simulink model "FIR_Filter"  (R2023b)
settings: Solver=FixedStepDiscrete  StartTime=0.0  StopTime=0.01  RelTol=1e-3
PreLoadFcn:
  | addpath('D:\Digital IC\FPGA\fir_filter\verif\hdlimport\FIR_Filter');
libraries: hdlmdlgenlib x60, dspsrcs4 x2
CloseFcn:
  | addpath('D:\Digital IC\FPGA\fir_filter\verif\hdlimport\FIR_Filter');
  | rmpath('D:\Digital IC\FPGA\fir_filter\verif\hdlimport\FIR_Filter');
settings Model: DataTypeOverride=Off  Creator=Abanoub Hanna  LastModifiedBy=Abanoub Hanna
settings OptimizationCC: BlockReduction=off  ConditionallyExecuteInputs=off  DefaultParameterBehavior=Inlined  InheritOutputTypeSmallerThanSingle=on
settings DebuggingCC: AlgebraicLoopMsg=error  InheritedTsInSrcMsg=none  SingleTaskRateTransMsg=error  ParameterPrecisionLossMsg=none
settings HardwareCC: ProdBitPerPointer=32  ProdBitPerSizeT=32  ProdBitPerPtrDiffT=32  ProdLargestAtomicFloat=None  ProdIntDivRoundTo=Undefined  ProdEndianess=Unspecified  ProdWordSize=32  ProdHWDeviceType=ASIC/FPGA->ASIC/FPGA  TargetBitPerPointer=64  TargetBitPerSizeT=64  TargetBitPerPtrDiffT=64  TargetLongLongMode=on  TargetIntDivRoundTo=Zero  TargetEndianess=LittleEndian  TargetWordSize=64  TargetHWDeviceType=Custom Processor->MATLAB Host Computer  ProdEqTarget=off

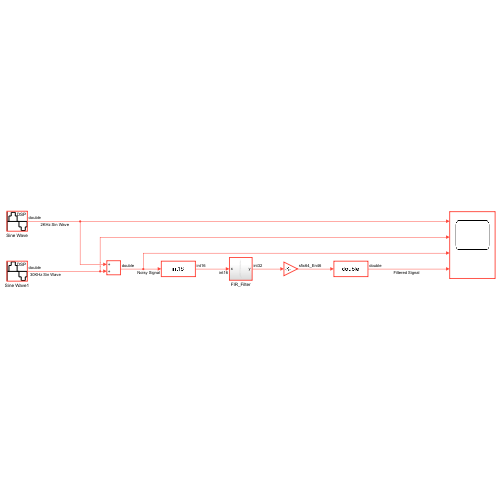
[thumbnail: Simulink's stored preview of the top-level diagram]
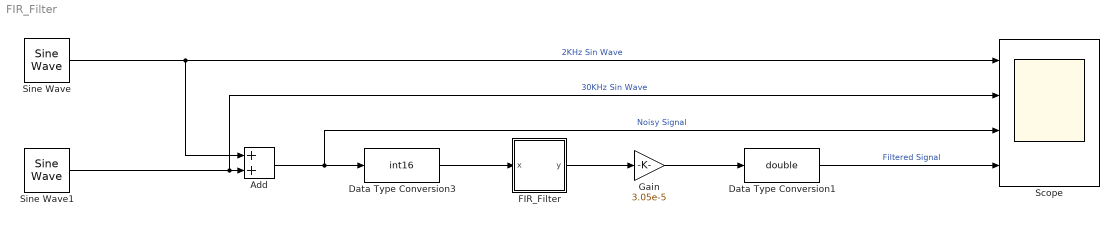
== system FIR_Filter ==
  Add : Sum  OutDataTypeStr=double
  Data Type Conversion1 : DataTypeConversion  OutDataTypeStr=double  RndMeth=Round  SaturateOnIntegerOverflow=off
  Data Type Conversion3 : DataTypeConversion  OutDataTypeStr=int16  RndMeth=Round  SaturateOnIntegerOverflow=off
  FIR_Filter : Subsystem
  Gain : Gain  Gain=3.05e-5
  Scope : Scope  NumInputPorts=4
  Sine Wave : dspsrcs4/Sine Wave  Amplitude=1  Frequency=2000  Phase=0  SampleMode=Discrete  OutComplex=Real  CompMethod=Trigonometric fcn  TableSize=Speed  SampleTime=1/100000  SamplesPerFrame=1  ResetState=Restart at time zero  OutputFrames=off  dataType=double  wordLen=16  udDataType=sfix(16)  fracBitsMode=Best precision  numFracBits=15  OutDataTypeStr=double  LastOutDataTypeStr=double
  Sine Wave1 : dspsrcs4/Sine Wave  Amplitude=1  Frequency=30000  Phase=0  SampleMode=Discrete  OutComplex=Real  CompMethod=Trigonometric fcn  TableSize=Speed  SampleTime=1/100000  SamplesPerFrame=1  ResetState=Restart at time zero  OutputFrames=off  dataType=double  wordLen=16  udDataType=sfix(16)  fracBitsMode=Best precision  numFracBits=15  OutDataTypeStr=double  LastOutDataTypeStr=double
  wires:
  Sine Wave/1 -> Add/1, Scope/1  "2KHz Sin Wave"
  Add/1 -> Scope/3, Data Type Conversion3/1  "Noisy Signal"
  FIR_Filter/1(y) -> Gain/1
  Gain/1 -> Data Type Conversion1/1
  Data Type Conversion3/1 -> FIR_Filter/1(x)
  Data Type Conversion1/1 -> Scope/4  "Filtered Signal"
  Sine Wave1/1 -> Scope/2, Add/2  "30KHz Sin Wave"

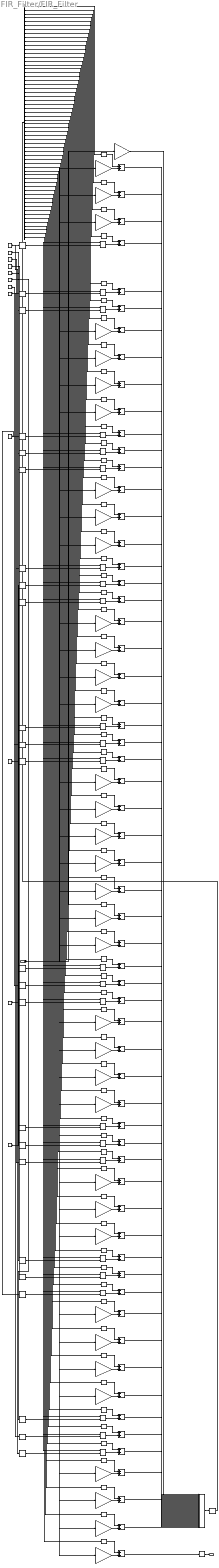
== system FIR_Filter/FIR_Filter ==
  x : Inport  OutDataTypeStr=int16  SampleTime=-1
  Add : Sum  OutDataTypeStr=int32  AccumDataTypeStr=int32  SampleTime=-1
  Add_{1..59} (59 alike) : Sum  OutDataTypeStr=int32  AccumDataTypeStr=int32  SampleTime=-1
  CONST_s32b_1479 : Constant  Value=1479  OutDataTypeStr=int32  SampleTime=-1
  CONST_s32b_168 : Constant  Value=168  OutDataTypeStr=int32  SampleTime=-1
  CONST_s32b_184 : Constant  Value=184  OutDataTypeStr=int32  SampleTime=-1
  CONST_s32b_1973 : Constant  Value=1973  OutDataTypeStr=int32  SampleTime=-1
  CONST_s32b_252 : Constant  Value=252  OutDataTypeStr=int32  SampleTime=-1
  CONST_s32b_36 : Constant  Value=36  OutDataTypeStr=int32  SampleTime=-1
  CONST_s32b_55 : Constant  Value=55  OutDataTypeStr=int32  SampleTime=-1
  CONST_s32b_582 : Constant  Value=582  OutDataTypeStr=int32  SampleTime=-1
  CONST_s32b_594 : Constant  Value=594  OutDataTypeStr=int32  SampleTime=-1
  CONST_s32b_77 : Constant  Value=77  OutDataTypeStr=int32  SampleTime=-1
  CONST_s32b_943 : Constant  Value=943  OutDataTypeStr=int32  SampleTime=-1
  CONST_s32b_95 : Constant  Value=95  OutDataTypeStr=int32  SampleTime=-1
  Mul{79,127,559,607} (4 alike) : Gain  Gain="fi(0,1,32,0,\"hex\",\"00000023\")"  ParamDataTypeStr=fixdt(1, 32, 0)  OutDataTypeStr=int32  SampleTime=-1
  Mul136 : Gain  Gain="fi(0,1,32,0,\"hex\",\"00000083\")"  ParamDataTypeStr=fixdt(1, 32, 0)  OutDataTypeStr=int32  SampleTime=-1
  Mul145 : Gain  Gain="fi(0,1,32,0,\"hex\",\"00000085\")"  ParamDataTypeStr=fixdt(1, 32, 0)  OutDataTypeStr=int32  SampleTime=-1
  Mul{62,154,250,436,532,624} (6 alike) : Gain  Gain="fi(0,1,32,0,\"hex\",\"00000000\")"  ParamDataTypeStr=fixdt(1, 32, 0)  OutDataTypeStr=int32  SampleTime=-1
  Mul193 : Gain  Gain="fi(0,1,32,0,\"hex\",\"000000d1\")"  ParamDataTypeStr=fixdt(1, 32, 0)  OutDataTypeStr=int32  SampleTime=-1
  Mul202 : Gain  Gain="fi(0,1,32,0,\"hex\",\"0000019a\")"  ParamDataTypeStr=fixdt(1, 32, 0)  OutDataTypeStr=int32  SampleTime=-1
  Mul211 : Gain  Gain="fi(0,1,32,0,\"hex\",\"00000115\")"  ParamDataTypeStr=fixdt(1, 32, 0)  OutDataTypeStr=int32  SampleTime=-1
  Mul259 : Gain  Gain="fi(0,1,32,0,\"hex\",\"0000030d\")"  ParamDataTypeStr=fixdt(1, 32, 0)  OutDataTypeStr=int32  SampleTime=-1
  Mul268 : Gain  Gain="fi(0,1,32,0,\"hex\",\"00000432\")"  ParamDataTypeStr=fixdt(1, 32, 0)  OutDataTypeStr=int32  SampleTime=-1
  Mul277 : Gain  Gain="fi(0,1,32,0,\"hex\",\"0000019d\")"  ParamDataTypeStr=fixdt(1, 32, 0)  OutDataTypeStr=int32  SampleTime=-1
  Mul316 : Gain  Gain="fi(0,1,32,0,\"hex\",\"0000041d\")"  ParamDataTypeStr=fixdt(1, 32, 0)  OutDataTypeStr=int32  SampleTime=-1
  Mul325 : Gain  Gain="fi(0,1,32,0,\"hex\",\"00001334\")"  ParamDataTypeStr=fixdt(1, 32, 0)  OutDataTypeStr=int32  SampleTime=-1
  Mul334 : Gain  Gain="fi(0,1,32,0,\"hex\",\"000020e4\")"  ParamDataTypeStr=fixdt(1, 32, 0)  OutDataTypeStr=int32  SampleTime=-1
  Mul343 : Gain  Gain="fi(0,1,32,0,\"hex\",\"00002666\")"  ParamDataTypeStr=fixdt(1, 32, 0)  OutDataTypeStr=int32  SampleTime=-1
  Mul352 : Gain  Gain="fi(0,1,32,0,\"hex\",\"000020e4\")"  ParamDataTypeStr=fixdt(1, 32, 0)  OutDataTypeStr=int32  SampleTime=-1
  Mul361 : Gain  Gain="fi(0,1,32,0,\"hex\",\"00001334\")"  ParamDataTypeStr=fixdt(1, 32, 0)  OutDataTypeStr=int32  SampleTime=-1
  Mul370 : Gain  Gain="fi(0,1,32,0,\"hex\",\"0000041d\")"  ParamDataTypeStr=fixdt(1, 32, 0)  OutDataTypeStr=int32  SampleTime=-1
  Mul409 : Gain  Gain="fi(0,1,32,0,\"hex\",\"0000019d\")"  ParamDataTypeStr=fixdt(1, 32, 0)  OutDataTypeStr=int32  SampleTime=-1
  Mul418 : Gain  Gain="fi(0,1,32,0,\"hex\",\"00000432\")"  ParamDataTypeStr=fixdt(1, 32, 0)  OutDataTypeStr=int32  SampleTime=-1
  Mul427 : Gain  Gain="fi(0,1,32,0,\"hex\",\"0000030d\")"  ParamDataTypeStr=fixdt(1, 32, 0)  OutDataTypeStr=int32  SampleTime=-1
  Mul475 : Gain  Gain="fi(0,1,32,0,\"hex\",\"00000115\")"  ParamDataTypeStr=fixdt(1, 32, 0)  OutDataTypeStr=int32  SampleTime=-1
  Mul484 : Gain  Gain="fi(0,1,32,0,\"hex\",\"0000019a\")"  ParamDataTypeStr=fixdt(1, 32, 0)  OutDataTypeStr=int32  SampleTime=-1
  Mul493 : Gain  Gain="fi(0,1,32,0,\"hex\",\"000000d1\")"  ParamDataTypeStr=fixdt(1, 32, 0)  OutDataTypeStr=int32  SampleTime=-1
  Mul541 : Gain  Gain="fi(0,1,32,0,\"hex\",\"00000085\")"  ParamDataTypeStr=fixdt(1, 32, 0)  OutDataTypeStr=int32  SampleTime=-1
  Mul550 : Gain  Gain="fi(0,1,32,0,\"hex\",\"00000083\")"  ParamDataTypeStr=fixdt(1, 32, 0)  OutDataTypeStr=int32  SampleTime=-1
  Mul598 : Gain  Gain="fi(0,1,32,0,\"hex\",\"0000000f\")"  ParamDataTypeStr=fixdt(1, 32, 0)  OutDataTypeStr=int32  SampleTime=-1
  Mul616 : Gain  Gain="fi(0,1,32,0,\"hex\",\"00000016\")"  ParamDataTypeStr=fixdt(1, 32, 0)  OutDataTypeStr=int32  SampleTime=-1
  Mul70 : Gain  Gain="fi(0,1,32,0,\"hex\",\"00000016\")"  ParamDataTypeStr=fixdt(1, 32, 0)  OutDataTypeStr=int32  SampleTime=-1
  Mul88 : Gain  Gain="fi(0,1,32,0,\"hex\",\"0000000f\")"  ParamDataTypeStr=fixdt(1, 32, 0)  OutDataTypeStr=int32  SampleTime=-1
  Mul_{4..6,11..13,17..19,24..26,34..36,41..43,47..49,54..56} (24 alike) : Product  Inputs=**  OutDataTypeStr=int32  SampleTime=-1
  Uminus : UnaryMinus  SampleTime=-1
  Uminus_{1..23} (23 alike) : UnaryMinus  SampleTime=-1
  VectorConcat : Concatenate  NumInputs=60
  acc_FF_0_wire : hdlmdlgenlib/Buffer
  acc_FF_10_wire : hdlmdlgenlib/Buffer
  acc_FF_11_wire : hdlmdlgenlib/Buffer
  acc_FF_12_wire : hdlmdlgenlib/Buffer
  acc_FF_13_wire : hdlmdlgenlib/Buffer
  acc_FF_14_wire : hdlmdlgenlib/Buffer
  acc_FF_15_wire : hdlmdlgenlib/Buffer
  acc_FF_16_wire : hdlmdlgenlib/Buffer
  acc_FF_17_wire : hdlmdlgenlib/Buffer
  acc_FF_18_wire : hdlmdlgenlib/Buffer
  acc_FF_19_wire : hdlmdlgenlib/Buffer
  acc_FF_1_wire : hdlmdlgenlib/Buffer
  acc_FF_20_wire : hdlmdlgenlib/Buffer
  acc_FF_21_wire : hdlmdlgenlib/Buffer
  acc_FF_22_wire : hdlmdlgenlib/Buffer
  acc_FF_23_wire : hdlmdlgenlib/Buffer
  acc_FF_24_wire : hdlmdlgenlib/Buffer
  acc_FF_25_wire : hdlmdlgenlib/Buffer
  acc_FF_26_wire : hdlmdlgenlib/Buffer
  acc_FF_27_wire : hdlmdlgenlib/Buffer
  acc_FF_28_wire : hdlmdlgenlib/Buffer
  acc_FF_29_wire : hdlmdlgenlib/Buffer
  acc_FF_2_wire : hdlmdlgenlib/Buffer
  acc_FF_30_wire : hdlmdlgenlib/Buffer
  acc_FF_31_wire : hdlmdlgenlib/Buffer
  acc_FF_32_wire : hdlmdlgenlib/Buffer
  acc_FF_33_wire : hdlmdlgenlib/Buffer
  acc_FF_34_wire : hdlmdlgenlib/Buffer
  acc_FF_35_wire : hdlmdlgenlib/Buffer
  acc_FF_36_wire : hdlmdlgenlib/Buffer
  acc_FF_37_wire : hdlmdlgenlib/Buffer
  acc_FF_38_wire : hdlmdlgenlib/Buffer
  acc_FF_39_wire : hdlmdlgenlib/Buffer
  acc_FF_3_wire : hdlmdlgenlib/Buffer
  acc_FF_40_wire : hdlmdlgenlib/Buffer
  acc_FF_41_wire : hdlmdlgenlib/Buffer
  acc_FF_42_wire : hdlmdlgenlib/Buffer
  acc_FF_43_wire : hdlmdlgenlib/Buffer
  acc_FF_44_wire : hdlmdlgenlib/Buffer
  acc_FF_45_wire : hdlmdlgenlib/Buffer
  acc_FF_46_wire : hdlmdlgenlib/Buffer
  acc_FF_47_wire : hdlmdlgenlib/Buffer
  acc_FF_48_wire : hdlmdlgenlib/Buffer
  acc_FF_49_wire : hdlmdlgenlib/Buffer
  acc_FF_4_wire : hdlmdlgenlib/Buffer
  acc_FF_50_wire : hdlmdlgenlib/Buffer
  acc_FF_51_wire : hdlmdlgenlib/Buffer
  acc_FF_52_wire : hdlmdlgenlib/Buffer
  acc_FF_53_wire : hdlmdlgenlib/Buffer
  acc_FF_54_wire : hdlmdlgenlib/Buffer
  acc_FF_55_wire : hdlmdlgenlib/Buffer
  acc_FF_56_wire : hdlmdlgenlib/Buffer
  acc_FF_57_wire : hdlmdlgenlib/Buffer
  acc_FF_58_wire : hdlmdlgenlib/Buffer
  acc_FF_59_wire : hdlmdlgenlib/Buffer
  acc_FF_5_wire : hdlmdlgenlib/Buffer
  acc_FF_6_wire : hdlmdlgenlib/Buffer
  acc_FF_7_wire : hdlmdlgenlib/Buffer
  acc_FF_8_wire : hdlmdlgenlib/Buffer
  acc_FF_9_wire : hdlmdlgenlib/Buffer
  acc_reg : Delay  DelayLength=double(1)  InitialCondition=0  SampleTime=-1
  t : Demux  Outputs=60
  y_1_reg : Delay  DelayLength=double(1)  InitialCondition=0  SampleTime=-1
  y : Outport  OutDataTypeStr=int32  SampleTime=-1
  wires:
  t/2 -> acc_FF_1_wire/1
  Mul_41/1 -> Add_40/2
  t/56 -> acc_FF_55_wire/1
  Add_25/1 -> VectorConcat/27
  acc_FF_32_wire/1 -> Add_32/1
  t/57 -> acc_FF_56_wire/1
  Uminus_18/1 -> Mul_47/2
  Mul418/1 -> Add_37/2
  Add_54/1 -> VectorConcat/56
  Mul_25/1 -> Add_24/2
  t/10 -> acc_FF_9_wire/1
  acc_FF_47_wire/1 -> Add_47/1
  Add_10/1 -> VectorConcat/12
  Mul277/1 -> Add_22/2
  t/59 -> acc_FF_58_wire/1
  t/4 -> acc_FF_3_wire/1
  Mul624/1 -> Add_59/2
  t/52 -> acc_FF_51_wire/1
  t/3 -> acc_FF_2_wire/1
  t/58 -> acc_FF_57_wire/1
  t/60 -> acc_FF_59_wire/1
  Mul_49/1 -> Add_48/2
  t/5 -> acc_FF_4_wire/1
  acc_FF_59_wire/1 -> Add_59/1
  CONST_s32b_36/1 -> Uminus/1, Uminus_23/1
  Add_13/1 -> VectorConcat/15
  t/18 -> acc_FF_17_wire/1
  Add_58/1 -> VectorConcat/60
  t/54 -> acc_FF_53_wire/1
  t/1 -> acc_FF_0_wire/1
  CONST_s32b_55/1 -> Uminus_21/1, Uminus_2/1
  t/55 -> acc_FF_54_wire/1
  Mul343/1 -> Add_29/2
  t/53 -> acc_FF_52_wire/1
  acc_FF_9_wire/1 -> Add_9/1
  Mul370/1 -> Add_32/2
  acc_FF_39_wire/1 -> Add_39/1
  Mul_18/1 -> Add_17/2
  t/35 -> acc_FF_34_wire/1
  Mul334/1 -> Add_28/2
  acc_FF_41_wire/1 -> Add_41/1
  t/51 -> acc_FF_50_wire/1
  Add_26/1 -> VectorConcat/28
  acc_reg/1 -> t/1
  Mul_56/1 -> Add_55/2
  x/1 -> Mul62/1, Mul624/1, Mul616/1, Mul_55/1, Mul_54/1, Mul541/1, Mul532/1, Mul475/1, Mul_43/1, Mul559/1, Mul436/1, Mul427/1, Mul409/1, Mul_36/1, Mul_34/1, Mul370/1, Mul_48/1, Mul361/1, Mul352/1, Mul343/1, Mul325/1, Mul316/1, Mul_26/1, Mul_25/1, Mul_24/1, Mul268/1, Mul259/1, Mul250/1, Mul_19/1, Mul_18/1, Mul_17/1, Mul211/1, Mul202/1, Mul193/1, Mul_12/1, Mul_11/1, Mul145/1, Mul127/1, Mul_6/1, Mul_5/1, Mul_4/1, Mul88/1, Mul79/1, Mul70/1, Mul607/1, Mul550/1, Mul_56/1, Mul_41/1, Mul154/1, Mul484/1, Mul_47/1, Mul277/1, Mul598/1, Mul_42/1, Mul334/1, Mul136/1, Mul493/1, Mul_49/1, Mul_13/1, Mul_35/1, Mul418/1
  Add_44/1 -> VectorConcat/46
  acc_FF_24_wire/1 -> Add_24/1
  Uminus_4/1 -> Mul_12/2
  Uminus_11/1 -> Mul_26/2
  t/50 -> acc_FF_49_wire/1
  t/48 -> acc_FF_47_wire/1
  t/49 -> acc_FF_48_wire/1
  t/47 -> acc_FF_46_wire/1
  Add_57/1 -> VectorConcat/59
  Add_16/1 -> VectorConcat/18
  CONST_s32b_943/1 -> Uminus_9/1, Uminus_14/1
  t/7 -> acc_FF_6_wire/1
  Uminus_6/1 -> Mul_17/2
  t/46 -> acc_FF_45_wire/1
  acc_FF_43_wire/1 -> Add_43/1
  t/19 -> acc_FF_18_wire/1
  Mul_42/1 -> Add_41/2
  t/34 -> acc_FF_33_wire/1
  acc_FF_30_wire/1 -> Add_30/1
  t/45 -> acc_FF_44_wire/1
  Add_8/1 -> VectorConcat/10
  t/44 -> acc_FF_43_wire/1
  t/42 -> acc_FF_41_wire/1
  acc_FF_46_wire/1 -> Add_46/1
  Uminus_13/1 -> Mul_35/2
  Mul475/1 -> Add_43/2
  t/43 -> acc_FF_42_wire/1
  Mul_4/1 -> Add_3/2
  t/41 -> acc_FF_40_wire/1
  CONST_s32b_1479/1 -> Uminus_12/1, Uminus_11/1
  Mul70/1 -> Add/2
  t/40 -> acc_FF_39_wire/1
  Mul259/1 -> Add_20/2
  t/39 -> acc_FF_38_wire/1
  t/38 -> acc_FF_37_wire/1
  t/37 -> acc_FF_36_wire/1
  Uminus/1 -> Mul_4/2
  t/36 -> acc_FF_35_wire/1
  acc_FF_35_wire/1 -> Add_35/1
  Uminus_15/1 -> Mul_41/2
  t/9 -> acc_FF_8_wire/1
  CONST_s32b_594/1 -> Uminus_16/1, Uminus_7/1
  t/25 -> acc_FF_24_wire/1
  y_1_reg/1 -> y/1
  Add_43/1 -> VectorConcat/45
  t/33 -> acc_FF_32_wire/1
  t/20 -> acc_FF_19_wire/1
  t/32 -> acc_FF_31_wire/1
  t/31 -> acc_FF_30_wire/1
  t/27 -> acc_FF_26_wire/1
  Add_12/1 -> VectorConcat/14
  t/30 -> acc_FF_29_wire/1
  t/29 -> acc_FF_28_wire/1
  t/28 -> acc_FF_27_wire/1
  t/21 -> acc_FF_20_wire/1
  t/24 -> acc_FF_23_wire/1
  Add_2/1 -> VectorConcat/4
  t/26 -> acc_FF_25_wire/1
  t/23 -> acc_FF_22_wire/1
  acc_FF_49_wire/1 -> Add_49/1
  Add/1 -> VectorConcat/2
  CONST_s32b_184/1 -> Uminus_20/1, Uminus_3/1
  acc_FF_13_wire/1 -> Add_13/1
  t/22 -> acc_FF_21_wire/1
  t/6 -> acc_FF_5_wire/1
  Add_37/1 -> VectorConcat/39
  t/15 -> acc_FF_14_wire/1
  t/17 -> acc_FF_16_wire/1
  t/16 -> acc_FF_15_wire/1
  acc_FF_55_wire/1 -> Add_55/1
  t/14 -> acc_FF_13_wire/1
  Add_22/1 -> VectorConcat/24
  t/13 -> acc_FF_12_wire/1
  t/12 -> acc_FF_11_wire/1
  t/11 -> acc_FF_10_wire/1
  Mul202/1 -> Add_14/2
  t/8 -> acc_FF_7_wire/1
  Add_59/1 -> y_1_reg/1
  Mul616/1 -> Add_58/2
  acc_FF_22_wire/1 -> Add_22/1
  Mul_34/1 -> Add_33/2
  Mul_26/1 -> Add_25/2
  Mul_12/1 -> Add_11/2
  Mul607/1 -> Add_57/2
  Add_56/1 -> VectorConcat/58
  Mul_55/1 -> Add_54/2
  Add_35/1 -> VectorConcat/37
  Mul598/1 -> Add_56/2
  Add_55/1 -> VectorConcat/57
  Mul532/1 -> Add_49/2
  Uminus_23/1 -> Mul_56/2
  Uminus_22/1 -> Mul_55/2
  Add_53/1 -> VectorConcat/55
  Mul_54/1 -> Add_53/2
  Uminus_21/1 -> Mul_54/2
  Uminus_14/1 -> Mul_36/2
  Add_52/1 -> VectorConcat/54
  acc_FF_31_wire/1 -> Add_31/1
  Mul559/1 -> Add_52/2
  Add_51/1 -> VectorConcat/53
  Mul_43/1 -> Add_42/2
  Mul550/1 -> Add_51/2
  Add_50/1 -> VectorConcat/52
  acc_FF_29_wire/1 -> Add_29/1
  Mul541/1 -> Add_50/2
  Add_49/1 -> VectorConcat/51
  Add_48/1 -> VectorConcat/50
  CONST_s32b_252/1 -> Uminus_4/1, Uminus_19/1
  Uminus_20/1 -> Mul_49/2
  Add_47/1 -> VectorConcat/49
  Mul_48/1 -> Add_47/2
  acc_FF_52_wire/1 -> Add_52/1
  Uminus_19/1 -> Mul_48/2
  Add_46/1 -> VectorConcat/48
  Mul_47/1 -> Add_46/2
  Add_45/1 -> VectorConcat/47
  Mul493/1 -> Add_45/2
  acc_FF_28_wire/1 -> Add_28/1
  Mul484/1 -> Add_44/2
  Uminus_3/1 -> Mul_11/2
  Add_42/1 -> VectorConcat/44
  Uminus_17/1 -> Mul_43/2
  Add_41/1 -> VectorConcat/43
  Uminus_16/1 -> Mul_42/2
  acc_FF_51_wire/1 -> Add_51/1
  Add_40/1 -> VectorConcat/42
  Add_39/1 -> VectorConcat/41
  acc_FF_21_wire/1 -> Add_21/1
  Mul436/1 -> Add_39/2
  Mul_17/1 -> Add_16/2
  Add_38/1 -> VectorConcat/40
  acc_FF_33_wire/1 -> Add_33/1
  Mul427/1 -> Add_38/2
  Add_36/1 -> VectorConcat/38
  Mul409/1 -> Add_36/2
  Mul_36/1 -> Add_35/2
  acc_FF_8_wire/1 -> Add_8/1
  Add_34/1 -> VectorConcat/36
  Mul_35/1 -> Add_34/2
  Add_33/1 -> VectorConcat/35
  Uminus_12/1 -> Mul_34/2
  Add_32/1 -> VectorConcat/34
  Add_31/1 -> VectorConcat/33
  Mul361/1 -> Add_31/2
  Add_30/1 -> VectorConcat/32
  acc_FF_2_wire/1 -> Add_2/1
  Mul352/1 -> Add_30/2
  Add_29/1 -> VectorConcat/31
  Add_28/1 -> VectorConcat/30
  Add_27/1 -> VectorConcat/29
  Mul325/1 -> Add_27/2
  Mul316/1 -> Add_26/2
  Mul88/1 -> Add_2/2
  Add_14/1 -> VectorConcat/16
  Add_24/1 -> VectorConcat/26
  Uminus_10/1 -> Mul_25/2
  Mul127/1 -> Add_6/2
  Mul145/1 -> Add_8/2
  Add_23/1 -> VectorConcat/25
  Mul_24/1 -> Add_23/2
  Uminus_9/1 -> Mul_24/2
  acc_FF_54_wire/1 -> Add_54/1
  Add_21/1 -> VectorConcat/23
  Mul268/1 -> Add_21/2
  Add_20/1 -> VectorConcat/22
  Add_19/1 -> VectorConcat/21
  Mul250/1 -> Add_19/2
  Add_18/1 -> VectorConcat/20
  Mul211/1 -> Add_15/2
  Mul_19/1 -> Add_18/2
  Uminus_8/1 -> Mul_19/2
  Add_17/1 -> VectorConcat/19
  Uminus_7/1 -> Mul_18/2
  acc_FF_36_wire/1 -> Add_36/1
  Add_15/1 -> VectorConcat/17
  CONST_s32b_582/1 -> Uminus_8/1, Uminus_15/1
  Mul193/1 -> Add_13/2
  Mul_13/1 -> Add_12/2
  VectorConcat/1 -> acc_reg/1
  Uminus_5/1 -> Mul_13/2
  CONST_s32b_95/1 -> Uminus_5/1, Uminus_18/1
  Add_11/1 -> VectorConcat/13
  Add_3/1 -> VectorConcat/5
  Mul_11/1 -> Add_10/2
  Add_9/1 -> VectorConcat/11
  Mul62/1 -> VectorConcat/1
  Mul154/1 -> Add_9/2
  CONST_s32b_1973/1 -> Uminus_10/1, Uminus_13/1
  Add_7/1 -> VectorConcat/9
  Mul136/1 -> Add_7/2
  Add_6/1 -> VectorConcat/8
  Add_5/1 -> VectorConcat/7
  Mul_6/1 -> Add_5/2
  Uminus_2/1 -> Mul_6/2
  Add_4/1 -> VectorConcat/6
  Mul_5/1 -> Add_4/2
  Uminus_1/1 -> Mul_5/2
  Add_1/1 -> VectorConcat/3
  Mul79/1 -> Add_1/2
  acc_FF_58_wire/1 -> Add_58/1
  acc_FF_57_wire/1 -> Add_57/1
  acc_FF_56_wire/1 -> Add_56/1
  acc_FF_53_wire/1 -> Add_53/1
  acc_FF_50_wire/1 -> Add_50/1
  acc_FF_48_wire/1 -> Add_48/1
  acc_FF_45_wire/1 -> Add_45/1
  acc_FF_44_wire/1 -> Add_44/1
  acc_FF_42_wire/1 -> Add_42/1
  acc_FF_40_wire/1 -> Add_40/1
  acc_FF_38_wire/1 -> Add_38/1
  acc_FF_18_wire/1 -> Add_18/1
  acc_FF_37_wire/1 -> Add_37/1
  acc_FF_34_wire/1 -> Add_34/1
  acc_FF_7_wire/1 -> Add_7/1
  acc_FF_27_wire/1 -> Add_27/1
  acc_FF_26_wire/1 -> Add_26/1
  acc_FF_25_wire/1 -> Add_25/1
  acc_FF_23_wire/1 -> Add_23/1
  acc_FF_20_wire/1 -> Add_20/1
  acc_FF_19_wire/1 -> Add_19/1
  acc_FF_17_wire/1 -> Add_17/1
  acc_FF_16_wire/1 -> Add_16/1
  acc_FF_15_wire/1 -> Add_15/1
  acc_FF_14_wire/1 -> Add_14/1
  acc_FF_12_wire/1 -> Add_12/1
  acc_FF_11_wire/1 -> Add_11/1
  acc_FF_10_wire/1 -> Add_10/1
  acc_FF_6_wire/1 -> Add_6/1
  acc_FF_5_wire/1 -> Add_5/1
  acc_FF_4_wire/1 -> Add_4/1
  acc_FF_3_wire/1 -> Add_3/1
  acc_FF_1_wire/1 -> Add_1/1
  acc_FF_0_wire/1 -> Add/1
  CONST_s32b_168/1 -> Uminus_17/1, Uminus_6/1
  CONST_s32b_77/1 -> Uminus_22/1, Uminus_1/1
